simulink model "lookupTableDynamic_TestGen35"  (R2017b)
settings: Solver=FixedStepDiscrete  StartTime=0.0  StopTime=10.0  RelTol=1e-3
libraries: simulink x1
settings Model: Creator=ktrinh  LastModifiedBy=ktrinh
settings DebuggingCC: ParameterOverflowMsg=none

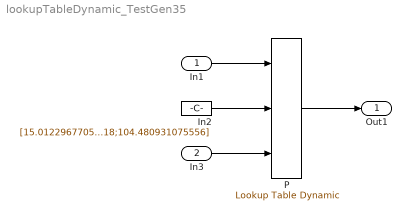
== system lookupTableDynamic_TestGen35 ==
  In1 : Inport  OutMin=13.0123  OutMax=106  OutDataTypeStr=int8  PortDimensions=[2,3]
  In3 : Inport  Port=2  PortDimensions=5
  In2 : Constant  Value=[15.0122967705343;36.0654679131294;68.0292034377719;69.4845102154118;104.480931075556]  OutDataTypeStr=int8
  P : simulink/Lookup Tables/Lookup Table Dynamic  LookUpMeth=Use Input Above  OutDataType=fixdt('uint32')  OutScaling=[]  OutputDataTypeScalingMode=Specify via dialog  OutDataTypeStr=uint32  RndMeth=Ceiling  DoSatur=on
      settings: SourceProductName=Simulink
  Out1 : Outport
  wires:
  In1/1 -> P/1
  In2/1 -> P/2
  In3/1 -> P/3
  P/1 -> Out1/1
